simulink model "Test_Case_2"  (R2017b)
settings: Solver=VariableStepAuto  StartTime=0.0  StopTime=inf  RelTol=1e-3
libraries: DigitalControlLib2 x4, simulink x1, realtime_pacer_lib x1
settings Model: Creator=alexandersoussan  LastModifiedBy=alexandersoussan

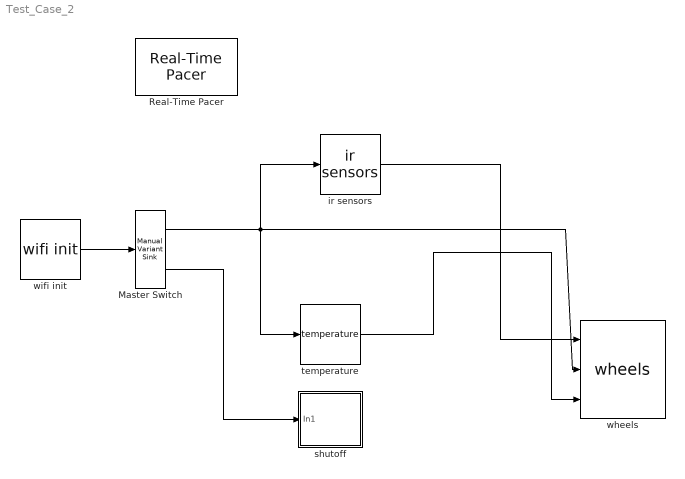
== system Test_Case_2 ==
  Master Switch : simulink/Signal Routing/Manual Variant Sink  NumChoices=2  OverrideUsingVariant=V_1
      settings: SourceProductName=Simulink
  Real-Time Pacer : realtime_pacer_lib/Real-Time Pacer  simTimePerRealTime=.5
  ir sensors : DigitalControlLib2/ir sensors
  shutoff : Subsystem
  temperature : DigitalControlLib2/temperature
  wheels : DigitalControlLib2/wheels
  wifi init : DigitalControlLib2/wifi init
  wires:
  ir sensors/1 -> wheels/1
  temperature/1 -> wheels/3
  wifi init/1 -> Master Switch/1
  Master Switch/1 -> ir sensors/1, temperature/1, wheels/2
  Master Switch/2 -> shutoff/1(In1)

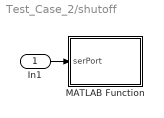
== system Test_Case_2/shutoff ==
  In1 : Inport
  MATLAB Function : MATLAB Function  TreatAsAtomicUnit=on
  wires:
  In1/1 -> MATLAB Function/1(serPort)

== matlab function Test_Case_2/shutoff/MATLAB Function ==
  data: serPort input
function PowerOffRoomba(serPort)
% PowerOffRoomba(serPort)
% Power down robot.  
% serPort is a serial port object created by RoombaInit
% Note that the physical power button does not work, and power saving and charging will not
% occur once the robot is initialized with RoombaInit.  There is a real
% risk of deeply discharging the Roomba's battery causing permanent
% damage.  Always use this command when done! 
% By Joel Esposito, US Naval Academy 2015
fwrite(serPort, [141 3]); % play RoombaInit song
pause(1);
fwrite(serPort, 133);
